simulink library "util_generic_model_lib"  (R2016b)
settings: Solver=ode45  StartTime=0.0  StopTime=10.0  RelTol=1e-3  EnableMultiTasking=on
undefined symbols (not defined in the file): abp_impeller_diameter, abp_impeller_speed2pwm, abp_nozzle_flap_count, abp_nozzle_flap_length, abp_nozzle_gear_ratio, abp_nozzle_intake_height, abp_nozzle_min_open_angle, abp_P_CG_B_B_error, abp_PM1_discharge_coeff, abp_pm1_impeller_orientation, abp_PM1_nozzle_orientations, abp_PM1_nozzle_widths, abp_PM1_P_nozzle_B_B, abp_pm1_zero_thrust_area, astrobee_time_step_size, bmp_PM1_impeller_orientation_error, bpm_imp_cmd_filt_den, bpm_imp_cmd_filt_num, bpm_imp_ctl_filt_n, bpm_imp_ctl_kd, bpm_imp_ctl_ki, bpm_imp_ctl_kp, bpm_imp_ctl_ts, bpm_imp_max_voltage, bpm_imp_motor_friction_coeff, bpm_imp_motor_r, bpm_imp_motor_speed_k, bpm_imp_motor_torque_k, bpm_imp_speed_filt_den, bpm_imp_speed_filt_num, bpm_impeller_inertia, bpm_impeller_inertia_error, bpm_impeller_init_speed, bpm_lookup_Cdp_data, bpm_lookup_totalarea_breakpoints, bpm_noise_on_flag, bpm_PM1_nozzle_discharge_coeff_error, bpm_PM1_nozzle_noise_feedback_gain, bpm_PM1_nozzle_thrust_noise_1s, bpm_PM1_P_nozzle_B_B_error, bpm_PM1_Q_nozzle2misaligned, bpm_PM1_randn_noise_seed, bpm_PM1_zero_thrust_area_error, bpm_sensor_delay, bpm_sensor_max, bpm_sensor_min, bpm_sensor_rand_seed, bpm_sensor_resolution, bpm_sensor_sf, bpm_sensor_sigma_u, bpm_sensor_sigma_v, bpm_servo_ctl_filt_n, bpm_servo_ctl_kd, bpm_servo_ctl_ki, bpm_servo_ctl_kp, bpm_servo_ctl_ts, bpm_servo_max_theta, bpm_servo_max_voltage, bpm_servo_min_theta, bpm_servo_motor_backlash_deadband ... (+45)
libraries: math_utils x8, simulink x4, vrlib x3, util_generic_model_lib x2
(part 1 of 2)
settings Model: Creator=rhnakamu  LastModifiedBy=jfusco1
settings DataIOCC: LimitDataPoints=on  SaveFormat=Array
settings OptimizationCC: LifeSpan=inf
settings DebuggingCC: AllowSymbolicDim=off  SFUnexpectedBacktrackingDiag=warning  SFNoUnconditionalDefaultTransitionDiag=warning  SFExecutionAtInitializationDiag=none
settings HardwareCC: ProdBitPerPointer=32  ProdBitPerSizeT=32  ProdBitPerPtrDiffT=32  ProdLargestAtomicFloat=None  ProdIntDivRoundTo=Undefined  ProdEndianess=Unspecified  ProdWordSize=32  ProdHWDeviceType=32-bit Generic
settings ModelReferenceCC: PropagateSignalLabelsOutOfModel=off
settings GRTTargetCC: TargetLangStandard=C89/C90 (ANSI)  GeneratePreprocessorConditionals=Disable all
settings ConfigComp: CovMetricSettings=dw  CovHtmlReporting=on  CovSaveCumulativeToWorkspaceVar=on  CovSaveSingleToWorkspaceVar=on  CovExternalEMLEnable=off

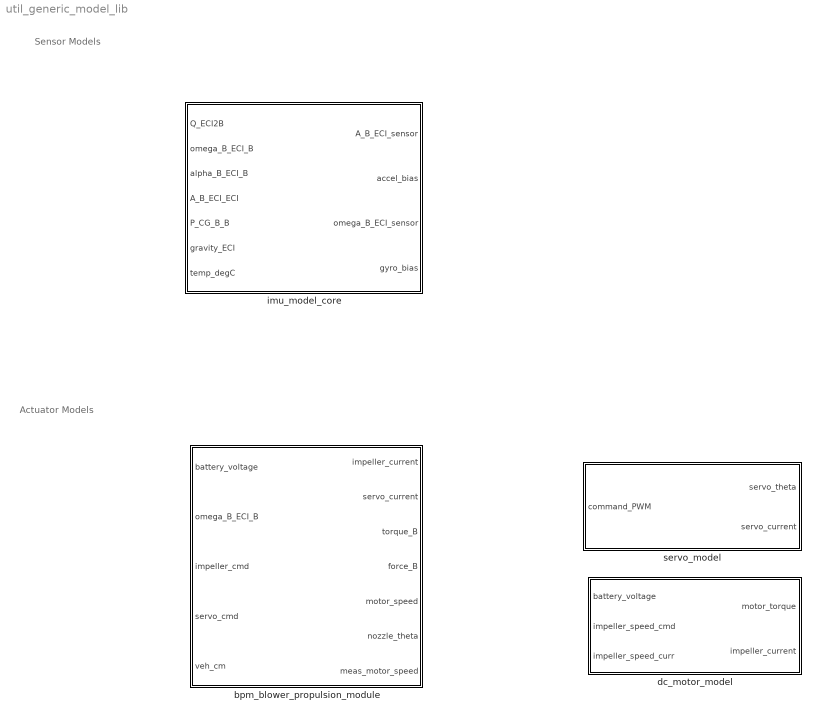
== system util_generic_model_lib ==
  note: Sensor Models
  note: Actuator Models
  bpm_blower_propulsion_module : Subsystem  mask{s_ctl_ts=bpm_servo_ctl_ts, s_ctl_pwm2angle=bpm_servo_pwm2angle, s_ctl_pwm2angle_bias=bpm_servo_pwm2angle_bias, s_ctl_kp=bpm_servo_ctl_kp, s_ctl_ki=bpm_servo_ctl_ki, s_ctl_kd=bpm_servo_ctl_kd, s_ctl_filt_n=bpm_servo_ctl_filt_n, s_ctl_max_volt=bpm_servo_max_voltage, s_motor_k=bpm_servo_motor_k, s_motor_r=bpm_servo_motor_r, s_motor_friction_coeff=bpm_servo_motor_friction_coeff, s_motor_gear_ratio=bpm_servo_motor_gear_ratio, s_motor_gear_box_inertia=bpm_servo_motor_gear_box_inertia, servo_max_theta=bpm_servo_max_theta, servo_min_theta=bpm_servo_min_theta, servo_backlash_deadband=bpm_servo_motor_backlash_deadband, P_nozzle_B_B=abp_PM1_P_nozzle_B_B, P_nozzle_B_B_offset=bpm_PM1_P_nozzle_B_B_error, nozzle_orientation_B=abp_PM1_nozzle_orientations, nozzle_orientation_offset=bpm_PM1_Q_nozzle2misaligned, noz_cd=abp_PM1_discharge_coeff, noz_cd_error=bpm_PM1_nozzle_discharge_coeff_error, noz_width=abp_PM1_nozzle_widths, noz_min_theta=abp_nozzle_min_open_angle, noz_intake_height=abp_nozzle_intake_height, noz_flap_length=abp_nozzle_flap_length, noz_flap_count=abp_nozzle_flap_count, noz_gear_ratio=abp_nozzle_gear_ratio, noz_thrust_noise=bpm_PM1_nozzle_thrust_noise_1s, noz_thrust_noise_feedback=bpm_PM1_nozzle_noise_feedback_gain, noz_randn_seed=bpm_PM1_randn_noise_seed, i_ctl_ts=bpm_imp_ctl_ts, i_ctl_pwm2speed=1/abp_impeller_speed2pwm, i_ctl_cmd_filt_num=bpm_imp_cmd_filt_num, i_ctl_cmd_filt_den=bpm_imp_cmd_filt_den, i_ctl_speed_filt_num=bpm_imp_speed_filt_num, i_ctl_speed_filt_den=bpm_imp_speed_filt_den, i_ctl_kp=bpm_imp_ctl_kp, i_ctl_ki=bpm_imp_ctl_ki, i_ctl_kd=bpm_imp_ctl_kd, i_ctl_filt_n=bpm_imp_ctl_filt_n, i_ctl_max_volt=bpm_imp_max_voltage, i_motor_kn=bpm_imp_motor_speed_k, i_motor_r=bpm_imp_motor_r, i_motor_kt=bpm_imp_motor_torque_k, i_motor_friction_coeff=bpm_imp_motor_friction_coeff, imp_unit_vec_B=abp_pm1_impeller_orientation, imp_unit_vec_B_offset=bmp_PM1_impeller_orientation_error, imp_zero_thrust_area=abp_pm1_zero_thrust_area, imp_zero_thrust_area_error=bpm_PM1_zero_thrust_area_error, imp_diameter=abp_impeller_diameter, imp_cdp_lookup=bpm_lookup_Cdp_data, imp_area_lookup=bpm_lookup_totalarea_breakpoints, imp_inertia=bpm_impeller_inertia, imp_inertia_error=bpm_impeller_inertia_error, imp_init_speed=bpm_impeller_init_speed, sens_sf=bpm_sensor_sf, sens_sigma_u=bpm_sensor_sigma_u, sens_sigma_v=bpm_sensor_sigma_v, sens_rand_seed=bpm_sensor_rand_seed, sens_resolution=bpm_sensor_resolution, sens_max=bpm_sensor_max, sens_min=bpm_sensor_min, sens_delay=bpm_sensor_delay, P_CG_B_B_error=abp_P_CG_B_B_error, const_air_den=const_air_density, sim_step_size=astrobee_time_step_size, noise_on_flag=bpm_noise_on_flag}
      mask prompts: s_ctl_ts "Controller Sample Time"; s_ctl_pwm2angle "PWM2Angle Conversion Gain"; s_ctl_pwm2angle_bias "PWM2Angle Conversion Bias"; s_ctl_kp "PID Controller - P gain"; s_ctl_ki "PID Controller - I gain"; s_ctl_kd "PID Controller - D gain"; s_ctl_filt_n "PID Controller - filter"; s_ctl_max_volt "Max Voltage Output"; s_motor_k "Speed Constant (k)"; s_motor_r "Resistance (r)"; s_motor_friction_coeff "Friction Coefficient"; s_motor_gear_ratio "Gear Ratio"; s_motor_gear_box_inertia "Gear Box Inertia"; servo_max_theta "Servo Max Theta"; servo_min_theta "Servo Min Theta"; servo_backlash_deadband "Backlash Deadband"; P_nozzle_B_B_offset "P_nozzle_B_B offset"; nozzle_orientation_B "Nozzle Orientation (B frame)"; nozzle_orientation_offset "Nozzle Orientation (offset)"; noz_cd "Discharge Coefficients"; noz_cd_error "Discharge Coefficients Error"; noz_width "Widths"; noz_min_theta "Min Theta"; noz_intake_height "Intake Height"; noz_flap_length "Flap Length"; noz_flap_count "Flap Count (per nozzle)"; noz_gear_ratio "Servo2Nozzle Gear Ratio"; noz_thrust_noise "Nozzle Thrust Noise (1-sigma)"; noz_thrust_noise_feedback "Nozzle Thrust Noise Feedback Gain"; noz_randn_seed "Nozzle Randn Seed"; i_ctl_ts "Controller Sample Time"; i_ctl_pwm2speed "PWM2Speed Conversion Gain"; i_ctl_cmd_filt_num "Speed Cmd Filter (Num)"; i_ctl_cmd_filt_den "Speed Cmd Filter (Den)"; i_ctl_speed_filt_num "Speed Filt (Num)"; i_ctl_speed_filt_den "Speed Filt (Den)"; i_ctl_kp "PID Controller - P gain"; i_ctl_ki "PID Controller - I Gain"; i_ctl_kd "PID Controller - D gain"; i_ctl_filt_n "PID Controller - filter"; i_ctl_max_volt "Max Voltage Output"; i_motor_kn "Speed Constant (kn)"; i_motor_r "Resistance (r)"; i_motor_kt "Torque Constant (kt)"; i_motor_friction_coeff "Friction Coefficient"; imp_unit_vec_B "Rotational Unit Vector (B frame)"; imp_unit_vec_B_offset "Rotational Unit Vector Offset"; imp_zero_thrust_area "Zero Thrust Area (Leakage)"; imp_zero_thrust_area_error "Zero Thrust Area Error"; imp_diameter "Diameter"; imp_cdp_lookup "Lookup Cdp data"; imp_area_lookup "Lookup totalarea breakpoints"; imp_inertia "Inertia"; imp_inertia_error "Inertia Error"; imp_init_speed "Initial Speed"; sens_sf "Scale Factor"; sens_sigma_u "Sigma U (noise)"; sens_sigma_v "Sigma V (noise)"; sens_rand_seed "Randn Seed"; sens_resolution "Resolution"; sens_max "Max Output"; sens_min "Min Output"; sens_delay "Output Delay"; P_CG_B_B_error "Position of CG error"; const_air_den "Air Density Constant"; sim_step_size "Simulation Step Size"; noise_on_flag "Noise On Flag (1=on, 0=off)"
      mask DialogControl DescGroupVar Prompt: Blower Propulsion Model Parameters
  dc_motor_model : Subsystem  mask{controller_sample_time=0, ctl_pwm2speed=0, ctl_cmd_filt_num=0, ctl_cmd_filt_den=0, ctl_speed_filt_num=0, ctl_speed_cilt_den=0, ctl_kp=0, ctl_ki=0, ctl_kd=0, ctl_filt_n=0, ctl_max_voltage=0, motor_kn=0, motor_r=0, motor_kt=0, motor_friction_coeff=0}
      mask prompts: controller_sample_time "Controller Sample Time"; ctl_pwm2speed "PWM2Speed Conversion Gain"; ctl_cmd_filt_num "Speed Cmd Filter (Num)"; ctl_cmd_filt_den "Speed Cmd Filter (Den)"; ctl_speed_filt_num "Speed Filter (Num)"; ctl_speed_cilt_den "Speed Filter (Den)"; ctl_kp "PID Controller - P Gain"; ctl_ki "PID Controller - I Gain"; ctl_kd "PID Controller - D Gain"; ctl_filt_n "PID Controller - filter"; ctl_max_voltage "Max Voltage Output"; motor_kn "Speed Constant (kn)"; motor_r "Resistance (r)"; motor_kt "Torque Constant (kt)"; motor_friction_coeff "Friction Coefficient"
      mask DialogControl DescGroupVar Prompt: Generic DC Motor Model
  imu_model_core : Subsystem  mask{Q_B2accel_nominal=epson_Q_B2accel, Q_B2accel_error=0, Q_B2gyro_nominal=epson_Q_B2gyro, Q_B2gyro_error=0, P_sensor_B_B_nominal=epson_P_sensor_B_B, P_sensor_B_B_error=0, imu_output_delay=epson_output_delay, sample_time=astrobee_time_step_size, report_imu_truth=epson_gyro_report_truth, no_rot_effects=epson_no_rot_effects, accel_sf=epson_accel_sf_coef, accel_nonlinear_coeff=epson_accel_nonlinearity_coeff, accel_temp_coeff=epson_accel_temp_bias_coeff, accel_sigma_vrw=epson_accel_sigma_v, accel_sigma_arw=epson_accel_sigma_u, accel_bias_ic=epson_accel_bias_ic, accel_sigma_markov=epson_accel_sigma_w, accel_markov_tau=epson_accel_markov_tau, accel_noise_seed=epson_accel_noise_seed, accel_filter_num=epson_accel_filt_num, accel_filter_den=epson_accel_filt_den, accel_resolution=epson_accel_resolution, accel_upper_sat=epson_accel_upper_sat, accel_lower_sat=epson_accel_lower_sat, gyro_sf=epson_gyro_sf_coef, gyro_accel_sensitivity=epson_gyro_linear_accel_bias_coeff, gyro_nonlinear_coeff=epson_gyro_nonlinearity_coeff, gyro_temp_coeff=epson_gyro_temp_bias_coeff, gyro_sigma_arw=epson_gyro_sigma_v, gyro_sigma_rrw=epson_gyro_sigma_u, gyro_bias_ic=epson_gyro_bias_ic, gyro_sigma_markov=epson_gyro_sigma_w, gyro_markov_tau=epson_gyro_markov_tau, gyro_noise_seed=epson_gyro_noise_seed, gyro_filter_num=epson_gyro_filt_num, gyro_filter_den=epson_gyro_filt_den, gyro_resolution=epson_gyro_resolution, gyro_upper_sat=epson_gyro_upper_sat, gyro_lower_sat=epson_gyro_lower_sat}
      mask prompts: Q_B2accel_nominal "Q_B2accel (nominal):"; Q_B2accel_error "Q_B2accel (errors):"; Q_B2gyro_nominal "Q_B2gyro (nominal):"; Q_B2gyro_error "Q_B2gyro (errors):"; P_sensor_B_B_nominal "P_sensor_B_B (nominal):"; P_sensor_B_B_error "P_sensor_B_B (error):"; imu_output_delay "Output Delay:"; sample_time "Sample Time:"; report_imu_truth "Report Truth Flag"; no_rot_effects "No Rot Effects Flag"; accel_sf "Scale Factor Coefficient:"; accel_nonlinear_coeff "Non Linearity Coefficient:"; accel_temp_coeff "Temperature Coefficient:"; accel_sigma_vrw "Velocity Random Walk Sigma (m/s^(3/2))"; accel_sigma_arw "Acceleration Random Walk Sigma (m/sec^(5/2))"; accel_bias_ic "Bias I.C."; accel_sigma_markov "Markov Random Drift ((m/s^2)/s)"; accel_markov_tau "Markov Tau constant"; accel_noise_seed "Random Number Seed"; accel_filter_num "Internal Filter Numerator (coefficients)"; accel_filter_den "Internal Filter Denominator (coefficients)"; accel_resolution "Resolution:"; accel_upper_sat "Upper Saturation:"; accel_lower_sat "Lower Saturation:"; gyro_sf "Scale Factor Coefficient:"; gyro_accel_sensitivity "Linear Accel Coefficient:"; gyro_nonlinear_coeff "Non Linearity Coefficient:"; gyro_temp_coeff "Temperature Coefficient:"; gyro_sigma_arw "Angular Random Walk Sigma (rad/sqrt(sec))"; gyro_sigma_rrw "Rate Random Walk Sigma (rad/sec^(3/2))"; gyro_bias_ic "Bias I.C."; gyro_sigma_markov "Markov Random Drift (deg/s)"; gyro_markov_tau "Markov Tau Constant"; gyro_noise_seed "Random Number Seed"; gyro_filter_num "Internal Filter Numerator (coefficients)"; gyro_filter_den "Internal Filter Denominator (coefficients)"; gyro_resolution "Resolution:"; gyro_upper_sat "Upper Saturation:"; gyro_lower_sat "Lower Saturation:"
      mask DialogControl DescTextVar Prompt: Properties for the generic IMU model.
      mask DialogControl Container25 Prompt: Debugging Properties
      mask DialogControl Control6 Prompt: Units are m/s^2 unless stated
      mask DialogControl Container17 Prompt: Scale Factor
      mask DialogControl Container19 Prompt: Bias Coefficients:
      mask DialogControl Container16 Prompt: Noise Parameters
      mask DialogControl Container18 Prompt: Hardware Properties
      mask DialogControl Control7 Prompt: Units are rad/sec unless stated
      mask DialogControl Container20 Prompt: Scale Factor:
      mask DialogControl Container21 Prompt: Bias Coefficients:
      mask DialogControl Container16_copy_copy Prompt: Noise Parameters
      mask DialogControl Container18_copy Prompt: Hardware Properties
  servo_model : Subsystem  TreatAsAtomicUnit=on  mask{controller_sample_time=0, servo_pwm2angle=0, servo_pwm2angle_bias=0, servo_ctl_kp=0, servo_ctl_ki=0, servo_ctl_kd=0, servo_ctl_filt_n=0, servo_ctl_ts=0, servo_max_voltage=0, motor_k=0, motor_r=0, motor_friction_coeff=0, motor_gear_ratio=0, motor_gear_box_inertia=0, servo_max_theta=0, servo_min_theta=0, motor_backlash_deadband=0}
      mask prompts: controller_sample_time "Controller Sample Time"; servo_pwm2angle "PWM2Angle Conversion Gain"; servo_pwm2angle_bias "PWM2Angle Conversion Bias"; servo_ctl_kp "PID Controller - P gain"; servo_ctl_ki "PID Controller - I gain"; servo_ctl_kd "PID Controller - D gain"; servo_ctl_filt_n "PID Controller - filter"; servo_ctl_ts "PID Controller - sample time"; servo_max_voltage "Max Voltage output"; motor_k "Speed Constant (k)"; motor_r "Resistance (r)"; motor_friction_coeff "Friction Coefficient"; motor_gear_ratio "Gear Ratio"; motor_gear_box_inertia "Gear Box Inertia"; servo_max_theta "Servo Max Theta"; servo_min_theta "Servo Min Theta"; motor_backlash_deadband "Backlash Deadband"
      mask DialogControl DescGroupVar Prompt: Generic Servo Model

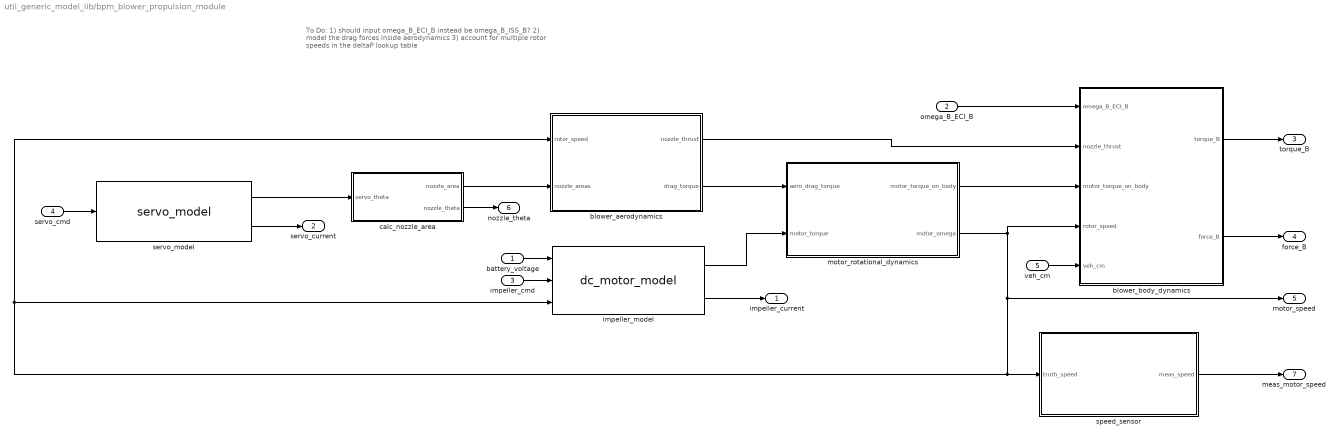
== system util_generic_model_lib/bpm_blower_propulsion_module ==
  note: To Do:
      | 	1) should input omega_B_ECI_B instead be omega_B_ISS_B?
      | 	2) model the drag forces inside aerodynamics
      | 	3) account for multiple rotor speeds in the deltaP lookup table
  battery_voltage : Inport
  omega_B_ECI_B : Inport  Port=2
  impeller_cmd : Inport  Port=3
  servo_cmd : Inport  Port=4
  veh_cm : Inport  Port=5
  blower_aerodynamics : Subsystem  TreatAsAtomicUnit=on  VariantControl=blw_blower_algebraic == true
      settings: RTWFcnNameOpts=Use subsystem name  RTWFileNameOpts=Use subsystem name
  blower_body_dynamics : Subsystem
  calc_nozzle_area : Subsystem  TreatAsAtomicUnit=on
  impeller_model : util_generic_model_lib/dc_motor_model  controller_sample_time=i_ctl_ts  ctl_pwm2speed=i_ctl_pwm2speed  ctl_cmd_filt_num=i_ctl_cmd_filt_num  ctl_cmd_filt_den=i_ctl_cmd_filt_den  ctl_speed_filt_num=i_ctl_speed_filt_num  ctl_speed_cilt_den=i_ctl_speed_filt_den  ctl_kp=i_ctl_kp  ctl_ki=i_ctl_ki  ctl_kd=i_ctl_kd  ctl_filt_n=i_ctl_filt_n  ctl_max_voltage=i_ctl_max_volt  motor_kn=i_motor_kn  motor_r=i_motor_r  motor_kt=i_motor_kt  motor_friction_coeff=i_motor_friction_coeff
  motor_rotational_dynamics : Subsystem
  servo_model : util_generic_model_lib/servo_model  controller_sample_time=s_ctl_ts  servo_pwm2angle=s_ctl_pwm2angle  servo_pwm2angle_bias=s_ctl_pwm2angle_bias  servo_ctl_kp=s_ctl_kp  servo_ctl_ki=s_ctl_ki  servo_ctl_kd=s_ctl_kd  servo_ctl_filt_n=s_ctl_filt_n  servo_ctl_ts=s_ctl_ts  servo_max_voltage=s_ctl_max_volt  motor_k=s_motor_k  motor_r=s_motor_r  motor_friction_coeff=s_motor_friction_coeff  motor_gear_ratio=s_motor_gear_ratio  motor_gear_box_inertia=s_motor_gear_box_inertia  servo_max_theta=servo_max_theta  servo_min_theta=servo_min_theta  motor_backlash_deadband=servo_backlash_deadband
  speed_sensor : Subsystem
  impeller_current : Outport
  servo_current : Outport  Port=2
  torque_B : Outport  Port=3
  force_B : Outport  Port=4
  motor_speed : Outport  Port=5
  nozzle_theta : Outport  Port=6
  meas_motor_speed : Outport  Port=7
  wires:
  blower_aerodynamics/1(nozzle_thrust) -> blower_body_dynamics/2(nozzle_thrust)
  battery_voltage/1 -> impeller_model/1
  calc_nozzle_area/1(nozzle_area) -> blower_aerodynamics/2(nozzle_areas)
  motor_rotational_dynamics/2(motor_omega) -> blower_body_dynamics/4(rotor_speed), motor_speed/1, impeller_model/3, blower_aerodynamics/1(rotor_speed), speed_sensor/1(truth_speed)
  servo_model/2 -> servo_current/1
  speed_sensor/1(meas_speed) -> meas_motor_speed/1
  omega_B_ECI_B/1 -> blower_body_dynamics/1(omega_B_ECI_B)
  servo_cmd/1 -> servo_model/1
  impeller_cmd/1 -> impeller_model/2
  impeller_model/1 -> motor_rotational_dynamics/2(motor_torque)
  impeller_model/2 -> impeller_current/1
  blower_aerodynamics/2(drag_torque) -> motor_rotational_dynamics/1(aero_drag_torque)
  motor_rotational_dynamics/1(motor_torque_on_body) -> blower_body_dynamics/3(motor_torque_on_body)
  servo_model/1 -> calc_nozzle_area/1(servo_theta)
  calc_nozzle_area/2(nozzle_theta) -> nozzle_theta/1
  blower_body_dynamics/1(torque_B) -> torque_B/1
  blower_body_dynamics/2(force_B) -> force_B/1
  veh_cm/1 -> blower_body_dynamics/5(veh_cm)

== system util_generic_model_lib/dc_motor_model ==
  battery_voltage : Inport
  impeller_speed_cmd : Inport  Port=2
  impeller_speed_curr : Inport  Port=3
  Rate Transition1 : RateTransition  OutPortSampleTime=controller_sample_time
      settings: AttributesFormatString=sampleTime: %<OutPortSampleTime>
  Rate Transition2 : RateTransition  OutPortSampleTime=controller_sample_time
      settings: AttributesFormatString=sampleTime: %<OutPortSampleTime>
  Rate Transition3 : RateTransition
      settings: AttributesFormatString=sampleTime: %<OutPortSampleTime>
  Rate Transition4 : RateTransition  OutPortSampleTime=controller_sample_time
      settings: AttributesFormatString=sampleTime: %<OutPortSampleTime>
  dc_motor_model : Subsystem  TreatAsAtomicUnit=on
  speed_controller : Subsystem  TreatAsAtomicUnit=on
  motor_torque : Outport
  impeller_current : Outport  Port=2
  wires:
  impeller_speed_curr/1 -> Rate Transition4/1, dc_motor_model/2(curr_rotor_speed)
  dc_motor_model/1(motor_torque) -> motor_torque/1
  speed_controller/1(motor_ctl_voltage) -> Rate Transition3/1
  dc_motor_model/2(motor_current) -> impeller_current/1
  battery_voltage/1 -> Rate Transition1/1
  Rate Transition3/1 -> dc_motor_model/1(ctl_voltage)
  Rate Transition1/1 -> speed_controller/1(battery_voltage)
  Rate Transition2/1 -> speed_controller/2(speed_cmd)
  Rate Transition4/1 -> speed_controller/3(speed_curr)
  impeller_speed_cmd/1 -> Rate Transition2/1

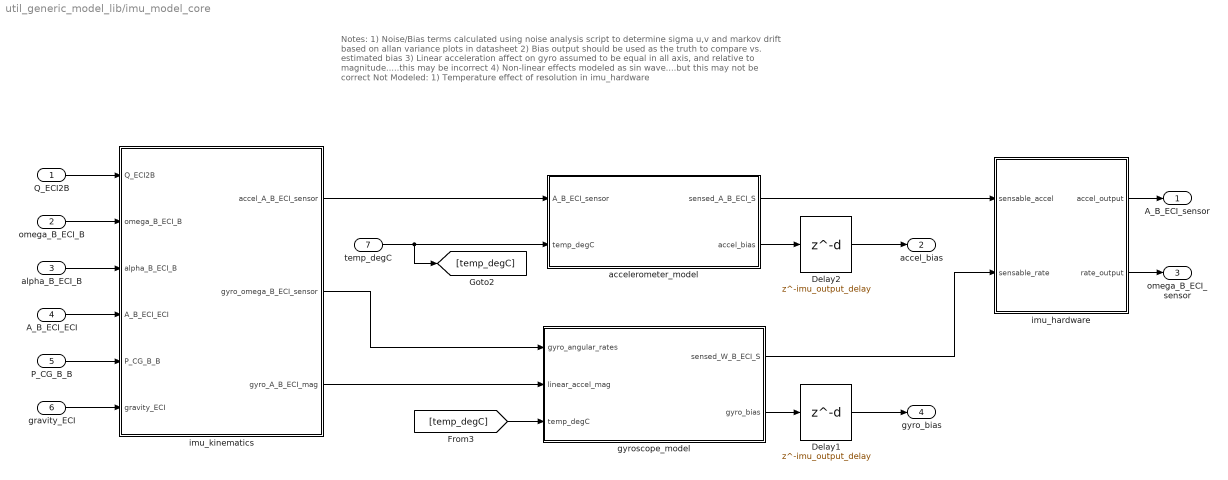
== system util_generic_model_lib/imu_model_core ==
  note: Notes:
      | 	1) Noise/Bias terms calculated using noise analysis script to determine sigma u,v and markov drift based on allan variance plots in datasheet
      | 	2) Bias output should be used as the truth to compare vs. estimated bias
      | 	3) Linear acceleration affect on gyro assumed to be equal in all axis, and relative to magnitude.....this may be incorrect
      | 	4) Non-linear effects modeled as sin wave....but this may not be correct
      |
      | Not Modeled:
      | 	1) Temperature effect of resolution in imu_hardware
  Q_ECI2B : Inport
  omega_B_ECI_B : Inport  Port=2
  alpha_B_ECI_B : Inport  Port=3
  A_B_ECI_ECI : Inport  Port=4
  P_CG_B_B : Inport  Port=5
  gravity_ECI : Inport  Port=6
  temp_degC : Inport  Port=7
  Delay1 : Delay  DelayLength=imu_output_delay
      settings: AttributesFormatString=|
      | IC: %<InitialCondition>
      | Delay: %<DelayLength>
  Delay2 : Delay  DelayLength=imu_output_delay
      settings: AttributesFormatString=|
      | IC: %<InitialCondition>
      | Delay: %<DelayLength>
  accelerometer_model : Subsystem
  gyroscope_model : Subsystem
  imu_hardware : Subsystem
  imu_kinematics : Subsystem
  A_B_ECI_sensor : Outport
  accel_bias : Outport  Port=2
  omega_B_ECI_sensor : Outport  Port=3
  gyro_bias : Outport  Port=4
  wires:
  omega_B_ECI_B/1 -> imu_kinematics/2(omega_B_ECI_B)
  imu_kinematics/2(gyro_omega_B_ECI_sensor) -> gyroscope_model/1(gyro_angular_rates)
  Delay1/1 -> gyro_bias/1
  Delay2/1 -> accel_bias/1
  [temp_degC] -> gyroscope_model/3(temp_degC)
  temp_degC/1 -> accelerometer_model/2(temp_degC), [temp_degC]
  imu_kinematics/1(accel_A_B_ECI_sensor) -> accelerometer_model/1(A_B_ECI_sensor)
  imu_kinematics/3(gyro_A_B_ECI_mag) -> gyroscope_model/2(linear_accel_mag)
  accelerometer_model/1(sensed_A_B_ECI_S) -> imu_hardware/1(sensable_accel)
  gyroscope_model/1(sensed_W_B_ECI_S) -> imu_hardware/2(sensable_rate)
  alpha_B_ECI_B/1 -> imu_kinematics/3(alpha_B_ECI_B)
  Q_ECI2B/1 -> imu_kinematics/1(Q_ECI2B)
  A_B_ECI_ECI/1 -> imu_kinematics/4(A_B_ECI_ECI)
  P_CG_B_B/1 -> imu_kinematics/5(P_CG_B_B)
  gravity_ECI/1 -> imu_kinematics/6(gravity_ECI)
  imu_hardware/2(rate_output) -> omega_B_ECI_sensor/1
  imu_hardware/1(accel_output) -> A_B_ECI_sensor/1
  gyroscope_model/2(gyro_bias) -> Delay1/1
  accelerometer_model/2(accel_bias) -> Delay2/1

== system util_generic_model_lib/servo_model ==
  command_PWM : Inport
  Rate Transition1 : RateTransition  OutPortSampleTime=controller_sample_time
      settings: AttributesFormatString=sampleTime: %<OutPortSampleTime>
  Rate Transition2 : RateTransition  OutPortSampleTime=controller_sample_time
      settings: AttributesFormatString=sampleTime: %<OutPortSampleTime>
  Rate Transition3 : RateTransition
      settings: AttributesFormatString=sampleTime: %<OutPortSampleTime>
  Terminator : Terminator
  dc_motor_dynamics : Subsystem
  servo_controller : Subsystem
  servo_theta : Outport
  servo_current : Outport  Port=2
  wires:
  dc_motor_dynamics/1(servo_theta) -> Rate Transition2/1, servo_theta/1
  dc_motor_dynamics/2(servo_current) -> servo_current/1
  Rate Transition2/1 -> servo_controller/2(curr_servo_theta)
  Rate Transition1/1 -> servo_controller/1(command_PWM)
  Rate Transition3/1 -> dc_motor_dynamics/1(ctl_voltage)
  servo_controller/1(motor_ctl_voltage) -> Rate Transition3/1
  command_PWM/1 -> Rate Transition1/1
  dc_motor_dynamics/3(servo_torque) -> Terminator/1

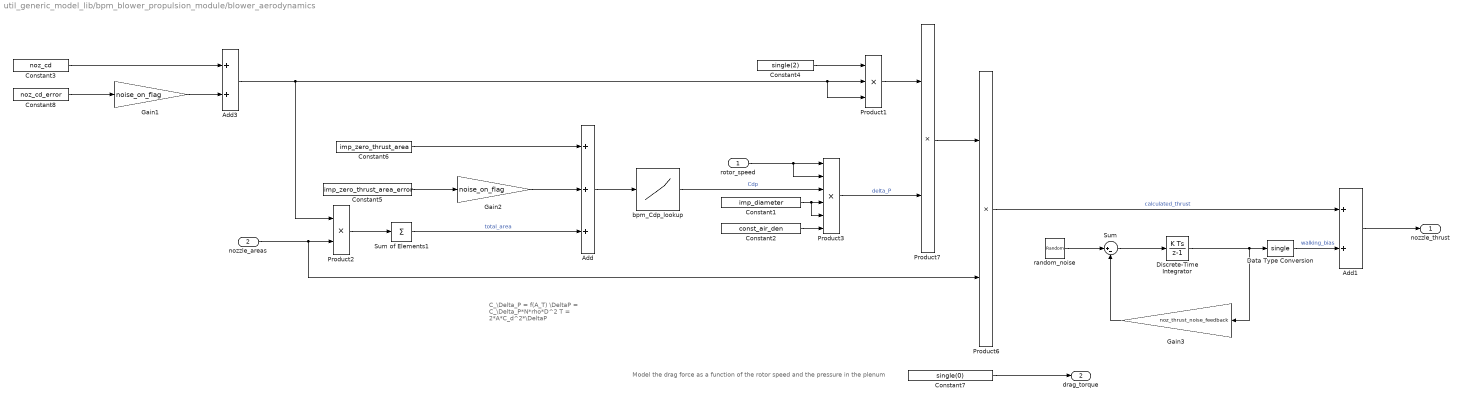
== system util_generic_model_lib/bpm_blower_propulsion_module/blower_aerodynamics ==
  note: Model the drag force as a function of the rotor speed and the pressure in the plenum
  note: C_\Delta_P = f(A_T)
      | \DeltaP = C_\Delta_P*N*rho*D^2
      | T = 2*A*C_d^2*\DeltaP
  rotor_speed : Inport
  nozzle_areas : Inport  Port=2
  Add : Sum  Inputs=+++
  Add1 : Sum
  Add3 : Sum
  Constant1 : Constant  Value=imp_diameter
  Constant2 : Constant  Value=const_air_den
  Constant3 : Constant  Value=noz_cd
  Constant4 : Constant  Value=single(2)
  Constant5 : Constant  Value=imp_zero_thrust_area_error
  Constant6 : Constant  Value=imp_zero_thrust_area
  Constant7 : Constant  Value=single(0)
  Constant8 : Constant  Value=noz_cd_error
  Data Type Conversion : DataTypeConversion  OutDataTypeStr=single
  Discrete-Time Integrator : DiscreteIntegrator  InitialConditionSetting=State (most efficient)  SampleTime=-1  ICPrevOutput=DiscIntNeverNeededParam  ICPrevScaledInput=DiscIntNeverNeededParam
      settings: AttributesFormatString=IC:%<InitialCondition>
  Gain1 : Gain  Gain=noise_on_flag
  Gain2 : Gain  Gain=noise_on_flag
  Gain3 : Gain  Gain=noz_thrust_noise_feedback
  Product1 : Product  Inputs=***
  Product2 : Product  Inputs=**
  Product3 : Product  Inputs=******
  Product6 : Product  Inputs=**
  Product7 : Product  Inputs=**
  Sum : Sum  Inputs=|+-
  Sum of Elements1 : Sum  Inputs=+
  bpm_Cdp_lookup : Lookup_n-D  NumberOfTableDimensions=1  BreakpointsForDimension1=imp_area_lookup  BreakpointsForDimension3=[5, 7]  Table=imp_cdp_lookup  InternalRulePriority=Speed  RndMeth=Simplest  InputSameDT=on
      settings: AttributesFormatString=|
      | data table: %<Table>
      | #dim: %<NumberOfTableDimensions>
      | BP1: %<BreakpointsForDimension1>
  random_noise : RandomNumber  Variance=noz_thrust_noise.^2  Seed=noz_randn_seed +[1:6]  SampleTime=sim_step_size
      settings: AttributesFormatString=|
      | Variance:%<Variance>
      | Mean:%<Mean>
      | Seed:%<Seed>
      | Sample Time:%<SampleTime>
  nozzle_thrust : Outport
  drag_torque : Outport  Port=2
  wires:
  Data Type Conversion/1 -> Add1/2  "walking_bias"
  Add1/1 -> nozzle_thrust/1
  Product6/1 -> Add1/1  "calculated_thrust"
  Gain3/1 -> Sum/2
  random_noise/1 -> Sum/1
  Sum/1 -> Discrete-Time Integrator/1
  Discrete-Time Integrator/1 -> Gain3/1, Data Type Conversion/1
  Constant2/1 -> Product3/6
  Product3/1 -> Product7/2  "delta_P"
  Constant1/1 -> Product3/5, Product3/4
  nozzle_areas/1 -> Product2/2, Product6/2
  Product1/1 -> Product7/1
  Constant4/1 -> Product1/1
  Add3/1 -> Product1/2, Product1/3, Product2/1
  bpm_Cdp_lookup/1 -> Product3/3  "Cdp"
  Sum of Elements1/1 -> Add/3  "total_area"
  rotor_speed/1 -> Product3/1, Product3/2
  Constant7/1 -> drag_torque/1
  Add/1 -> bpm_Cdp_lookup/1
  Constant6/1 -> Add/1
  Product2/1 -> Sum of Elements1/1
  Product7/1 -> Product6/1
  Constant8/1 -> Gain1/1
  Gain1/1 -> Add3/2
  Constant3/1 -> Add3/1
  Constant5/1 -> Gain2/1
  Gain2/1 -> Add/2

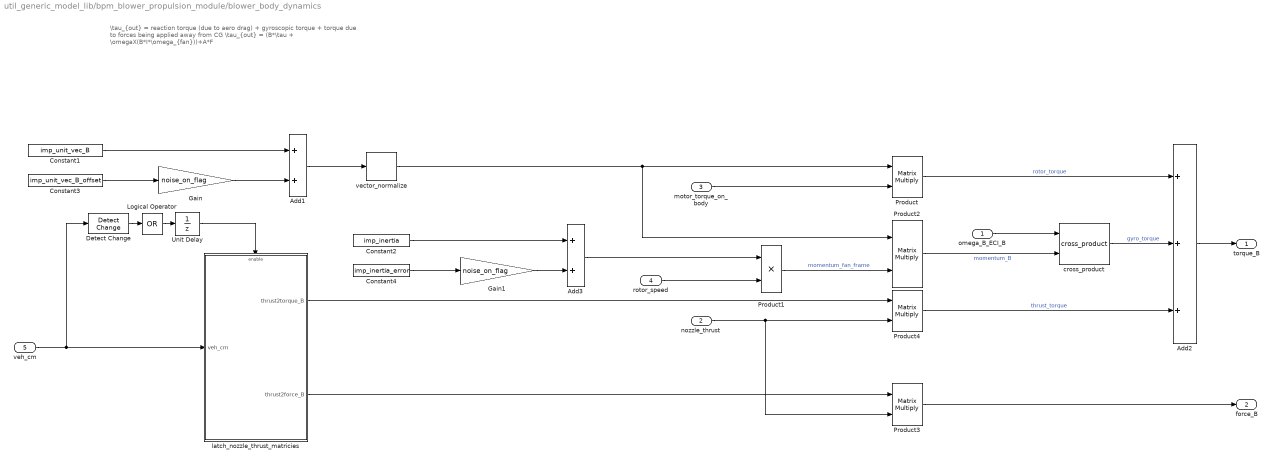
== system util_generic_model_lib/bpm_blower_propulsion_module/blower_body_dynamics ==
  note: \tau_{out} = reaction torque (due to aero drag)
      |                      + gyroscopic torque
      |                      + torque due to forces being applied away from CG
      | \tau_{out} = (B*\tau + \omegaX(B*I*\omega_{fan}))+A*F
  omega_B_ECI_B : Inport
  nozzle_thrust : Inport  Port=2
  motor_torque_on_body : Inport  Port=3
  rotor_speed : Inport  Port=4
  veh_cm : Inport  Port=5
  Add1 : Sum
  Add2 : Sum  Inputs=+++
  Add3 : Sum
  Constant1 : Constant  Value=imp_unit_vec_B
  Constant2 : Constant  Value=imp_inertia
  Constant3 : Constant  Value=imp_unit_vec_B_offset
  Constant4 : Constant  Value=imp_inertia_error
  Detect Change : simulink/Logic and Bit Operations/Detect Change  vinit=0  OutDataTypeStr=boolean
  Gain : Gain  Gain=noise_on_flag
  Gain1 : Gain  Gain=noise_on_flag
  Logical Operator : Logic  Operator=OR  Inputs=1  AllPortsSameDT=off  OutDataTypeStr=boolean
  Product{,2..4} (4 alike) : Product  Multiplication=Matrix(*)
  Product1 : Product
  Unit Delay : UnitDelay  InitialCondition=1  SampleTime=-1
      settings: AttributesFormatString=IC: %<InitialCondition>
  cross_product : math_utils/cross_product  SystemSampleTime=-1
  latch_nozzle_thrust_matricies : Subsystem
  vector_normalize : math_utils/vector_normalize  SystemSampleTime=-1
  torque_B : Outport
  force_B : Outport  Port=2
  wires:
  vector_normalize/1 -> Product2/1, Product/1
  Logical Operator/1 -> Unit Delay/1
  Unit Delay/1 -> latch_nozzle_thrust_matricies/Enable
  Product4/1 -> Add2/3  "thrust_torque"
  Product3/1 -> force_B/1
  nozzle_thrust/1 -> Product3/2, Product4/2
  Add2/1 -> torque_B/1
  cross_product/1 -> Add2/2  "gyro_torque"
  Product/1 -> Add2/1  "rotor_torque"
  Product2/1 -> cross_product/2  "momentum_B"
  omega_B_ECI_B/1 -> cross_product/1
  Product1/1 -> Product2/2  "momentum_fan_frame"
  Add1/1 -> vector_normalize/1
  rotor_speed/1 -> Product1/2
  motor_torque_on_body/1 -> Product/2
  Constant1/1 -> Add1/1
  Constant3/1 -> Gain/1
  Gain/1 -> Add1/2
  Constant4/1 -> Gain1/1
  Gain1/1 -> Add3/2
  Constant2/1 -> Add3/1
  Add3/1 -> Product1/1
  latch_nozzle_thrust_matricies/1(thrust2torque_B) -> Product4/1
  latch_nozzle_thrust_matricies/2(thrust2force_B) -> Product3/1
  veh_cm/1 -> Detect Change/1, latch_nozzle_thrust_matricies/1(veh_cm)
  Detect Change/1 -> Logical Operator/1

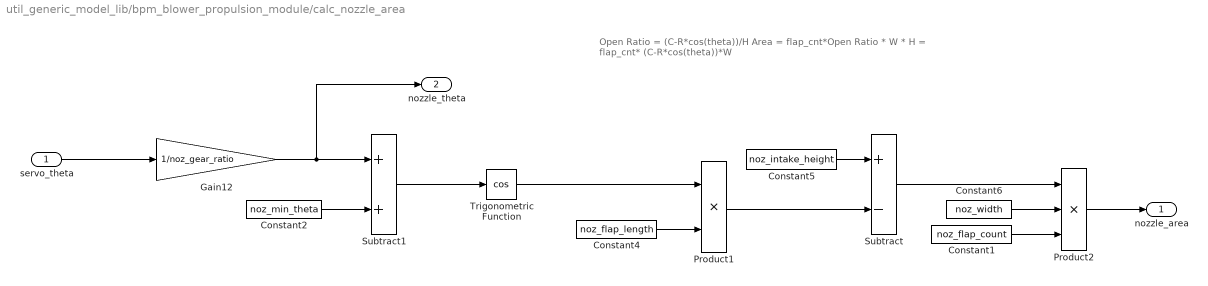
== system util_generic_model_lib/bpm_blower_propulsion_module/calc_nozzle_area ==
  note: Open Ratio = (C-R*cos(theta))/H
      |
      | Area = flap_cnt*Open Ratio * W * H = flap_cnt* (C-R*cos(theta))*W
  servo_theta : Inport
  Constant1 : Constant  Value=noz_flap_count
  Constant2 : Constant  Value=noz_min_theta
  Constant4 : Constant  Value=noz_flap_length
  Constant5 : Constant  Value=noz_intake_height
  Constant6 : Constant  Value=noz_width
  Gain12 : Gain  Gain=1/noz_gear_ratio
  Product1 : Product  Inputs=**
  Product2 : Product  Inputs=***
  Subtract : Sum  Inputs=+-
  Subtract1 : Sum
  Trigonometric Function : Trigonometry  Operator=cos
      settings: AttributesFormatString=Approx Method: %<ApproximationMethod>
  nozzle_area : Outport
  nozzle_theta : Outport  Port=2
  wires:
  Trigonometric Function/1 -> Product1/1
  Constant4/1 -> Product1/2
  Product1/1 -> Subtract/2
  Constant5/1 -> Subtract/1
  Subtract/1 -> Product2/1
  Constant6/1 -> Product2/2
  Constant1/1 -> Product2/3
  Subtract1/1 -> Trigonometric Function/1
  Product2/1 -> nozzle_area/1
  Constant2/1 -> Subtract1/2
  Gain12/1 -> Subtract1/1, nozzle_theta/1
  servo_theta/1 -> Gain12/1

== system util_generic_model_lib/bpm_blower_propulsion_module/motor_rotational_dynamics ==
  note: \tau_{total} = J*\omega' = \tau_{motor} -\tau_{drag} - \tau_{friction}
      |
      | Note: \tau_{friction} is accounted for in the motor model
  aero_drag_torque : Inport
  motor_torque : Inport  Port=2
  Add : Sum  Inputs=+-
  Constant : Constant  Value=noise_on_flag
  Discrete-Time Integrator : DiscreteIntegrator  InitialCondition=imp_init_speed  SampleTime=sim_step_size  ICPrevOutput=DiscIntNeverNeededParam  ICPrevScaledInput=DiscIntNeverNeededParam
      settings: AttributesFormatString=|
      | IC: %<InitialCondition>
      | TS: %<SampleTime>
  Gain : Gain  Gain=1./imp_inertia
  Gain1 : Gain  Gain=-1
  Gain2 : Gain  Gain=1./(imp_inertia+imp_inertia_error)
  Switch : Switch  Criteria=u2 > Threshold
  motor_torque_on_body : Outport
  motor_omega : Outport  Port=2
  wires:
  Discrete-Time Integrator/1 -> motor_omega/1  "omega"
  Gain1/1 -> motor_torque_on_body/1  "torque_on_body_due_to_motor"
  Add/1 -> Gain/1, Gain2/1  "torque_on_motor"
  Switch/1 -> Discrete-Time Integrator/1  "omega_dot"
  motor_torque/1 -> Gain1/1, Add/1
  aero_drag_torque/1 -> Add/2
  Constant/1 -> Switch/2
  Gain/1 -> Switch/1
  Gain2/1 -> Switch/3

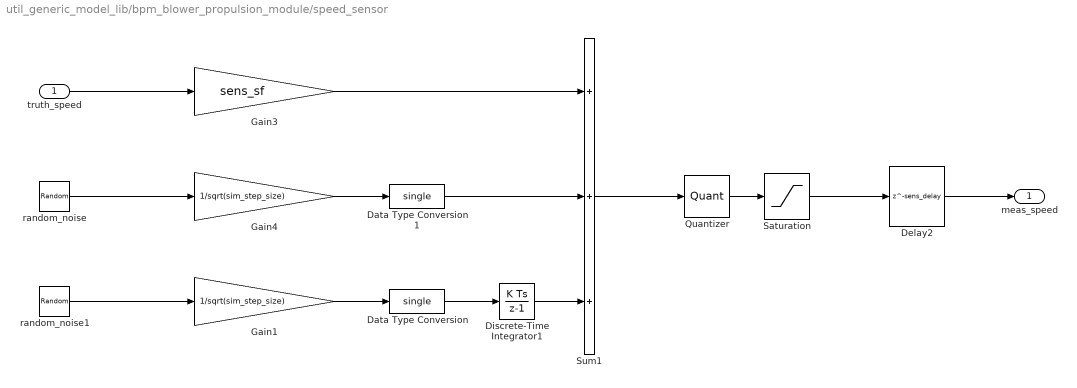
== system util_generic_model_lib/bpm_blower_propulsion_module/speed_sensor ==
  truth_speed : Inport
  Data Type Conversion : DataTypeConversion  OutDataTypeStr=single
  Data Type Conversion1 : DataTypeConversion  OutDataTypeStr=single
  Delay2 : Delay  DelayLength=sens_delay
      settings: AttributesFormatString=|
      | IC: %<InitialCondition>
      | Delay: %<DelayLength>
  Discrete-Time Integrator1 : DiscreteIntegrator  InitialCondition=single(0)  InitialConditionSetting=State (most efficient)  SampleTime=-1  ICPrevOutput=DiscIntNeverNeededParam  ICPrevScaledInput=DiscIntNeverNeededParam
      settings: AttributesFormatString=IC:%<InitialCondition>
  Gain1 : Gain  Gain=1/sqrt(sim_step_size)
  Gain3 : Gain  Gain=sens_sf
  Gain4 : Gain  Gain=1/sqrt(sim_step_size)
  Quantizer : Quantizer  QuantizationInterval=sens_resolution
  Saturation : Saturate  UpperLimit=sens_max  LowerLimit=sens_min
  Sum1 : Sum  Inputs=+++
  random_noise : RandomNumber  Variance=sens_sigma_u.^2  Seed=sens_rand_seed  SampleTime=sim_step_size
      settings: AttributesFormatString=|
      | Variance:%<Variance>
      | Mean:%<Mean>
      | Seed:%<Seed>
      | Sample Time:%<SampleTime>
  random_noise1 : RandomNumber  Variance=sens_sigma_v.^2  Seed=sens_rand_seed+1  SampleTime=sim_step_size
      settings: AttributesFormatString=|
      | Variance:%<Variance>
      | Mean:%<Mean>
      | Seed:%<Seed>
      | Sample Time:%<SampleTime>
  meas_speed : Outport
  wires:
  Data Type Conversion/1 -> Discrete-Time Integrator1/1
  Gain3/1 -> Sum1/1
  Data Type Conversion1/1 -> Sum1/2
  Discrete-Time Integrator1/1 -> Sum1/3
  Sum1/1 -> Quantizer/1
  Gain4/1 -> Data Type Conversion1/1
  Gain1/1 -> Data Type Conversion/1
  random_noise1/1 -> Gain1/1
  random_noise/1 -> Gain4/1
  truth_speed/1 -> Gain3/1
  Saturation/1 -> Delay2/1
  Delay2/1 -> meas_speed/1
  Quantizer/1 -> Saturation/1

== system util_generic_model_lib/dc_motor_model/dc_motor_model ==
  note: T_m = [(V- \omega*K_s)/R-i_o]*K_t - T_f
  note: Using negligible inductance formula from 'Comparison of Fixed and Variable Pitch Actuators for Agile Quadrotors'
  note: todo:
      | aero loading and dynamics
      | Stick-tion friction
  ctl_voltage : Inport
  curr_rotor_speed : Inport  Port=2
  Add : Sum  Inputs=+-
  Add1 : Sum  Inputs=+-
  Gain1 : Gain  Gain=motor_friction_coeff
  Gain4 : Gain  Gain=1/motor_kn
  Gain5 : Gain  Gain=1/motor_r
  Gain6 : Gain  Gain=motor_kt
  motor_torque : Outport
  motor_current : Outport  Port=2
  wires:
  Gain1/1 -> Add1/2  "viscous_friction"
  Add1/1 -> motor_torque/1  "output_torque"
  Gain6/1 -> Add1/1  "torque"
  Add/1 -> Gain5/1
  curr_rotor_speed/1 -> Gain4/1, Gain1/1
  Gain4/1 -> Add/2
  ctl_voltage/1 -> Add/1
  Gain5/1 -> motor_current/1, Gain6/1  "current"

== system util_generic_model_lib/dc_motor_model/speed_controller ==
  battery_voltage : Inport
  speed_cmd : Inport  Port=2
  speed_curr : Inport  Port=3
  Constant : Constant  Value=ctl_pwm2speed
  Discrete Transfer Fcn : DiscreteTransferFcn  Numerator=ctl_cmd_filt_num  Denominator=ctl_cmd_filt_den  SampleTime=controller_sample_time
      settings: AttributesFormatString=|
      | Num: %<Numerator>
      | Den: %<Denominator>
      | TS: %<SampleTime>
  Discrete Transfer Fcn1 : DiscreteTransferFcn  Numerator=ctl_speed_filt_num  Denominator=ctl_speed_cilt_den  SampleTime=controller_sample_time
      settings: AttributesFormatString=|
      | Num: %<Numerator>
      | Den: %<Denominator>
      | TS: %<SampleTime>
  Discrete PID Controller : simulink/Continuous/PID Controller  Controller=PID  TimeDomain=Discrete-time  SampleTime=controller_sample_time  IntegratorMethod=Forward Euler  FilterMethod=Forward Euler  Form=Parallel  UseFilter=on  ControllerParametersSource=internal  P=ctl_kp  I=ctl_ki  D=ctl_kd  N=ctl_filt_n  InitialConditionSource=internal  InitialConditionForIntegrator=0  InitialConditionForFilter=0  ExternalReset=none  LimitOutput=on  UpperSaturationLimit=ctl_max_voltage  LowerSaturationLimit=-ctl_max_voltage  LinearizeAsGain=off  AntiWindupMode=clamping  Kb=1  TrackingMode=off  Kt=1  PParamMin=[]  PParamMax=[]  IParamMin=[]  IParamMax=[]  DParamMin=[]  DParamMax=[]  NParamMin=[]  NParamMax=[]  KbParamMin=[]  KbParamMax=[]  KtParamMin=[]  KtParamMax=[]  POutMin=[]  POutMax=[]  IOutMin=[]  IOutMax=[]  DOutMin=[]  DOutMax=[]  NOutMin=[]  NOutMax=[]  KbOutMin=[]  KbOutMax=[]  KtOutMin=[]  KtOutMax=[]  IntegratorOutMin=[]  IntegratorOutMax=[]  FilterOutMin=[]  FilterOutMax=[]  SumOutMin=[]  SumOutMax=[]  SumI1OutMin=[]  SumI1OutMax=[]  SumI2OutMin=[]  SumI2OutMax=[]  SumI3OutMin=[]  SumI3OutMax=[]  SumDOutMin=[]  SumDOutMax=[]  SaturationOutMin=[]  SaturationOutMax=[]  IntegratorContinuousStateAttributes=''  IntegratorStateMustResolveToSignalObject=off  IntegratorRTWStateStorageClass=Auto  FilterContinuousStateAttributes=''  FilterStateMustResolveToSignalObject=off  FilterRTWStateStorageClass=Auto  DifferentiatorICPrevScaledInput=0  DifferentiatorOutMin=[]  DifferentiatorOutMax=[]
      settings: AttributesFormatString=|
      | Kp: %<P>
      | Ki: %<I>
      | Kd: %<D>
      | NFilt: %<N>
      | Ts: %<SampleTime>
      | 
      | min: %<LowerSaturationLimit>
      | max: %<UpperSaturationLimit>
  Divide : Product  Inputs=**
  Gain : Gain  Gain=-1
  Saturation Dynamic : simulink/Discontinuities/Saturation Dynamic  OutMin=[]  OutMax=[]  OutDataTypeStr=Inherit: Same as second input  OutDataType=fixdt(1, 16)  OutScaling=2^-10  DoSatur=off
  Sum : Sum  Inputs=+-
  motor_ctl_voltage : Outport
  wires:
  speed_cmd/1 -> Divide/1
  Constant/1 -> Divide/2
  Divide/1 -> Discrete Transfer Fcn/1
  Discrete Transfer Fcn/1 -> Sum/1
  Discrete Transfer Fcn1/1 -> Sum/2
  Saturation Dynamic/1 -> motor_ctl_voltage/1
  Sum/1 -> Discrete PID Controller/1
  speed_curr/1 -> Discrete Transfer Fcn1/1
  battery_voltage/1 -> Saturation Dynamic/1, [volt]
  Discrete PID Controller/1 -> Saturation Dynamic/2
  [volt] -> Gain/1
  Gain/1 -> Saturation Dynamic/3

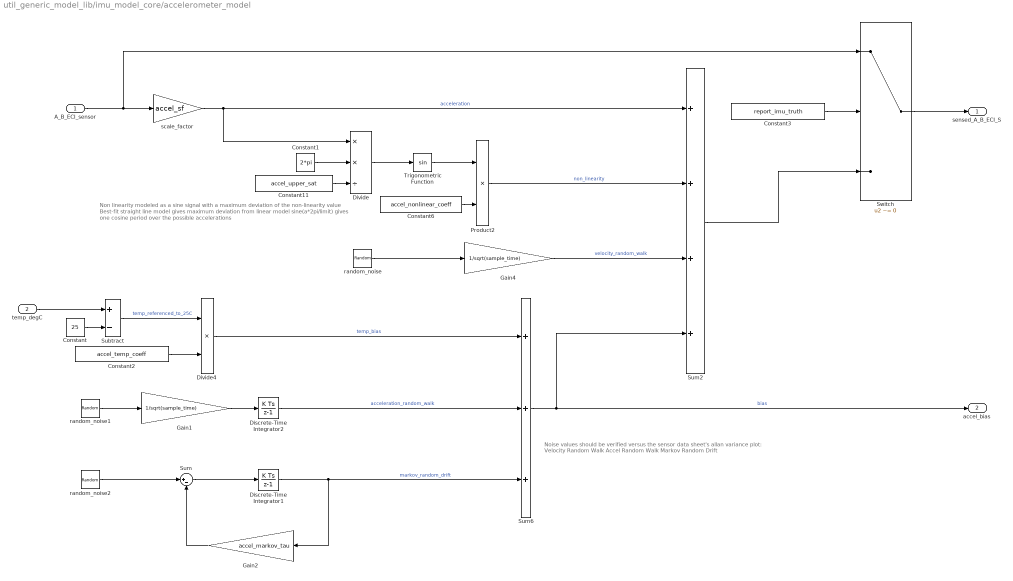
== system util_generic_model_lib/imu_model_core/accelerometer_model ==
  note: Non linearity modeled as a sine signal with a maximum deviation of the non-linearity value
      | Best-fit straight line model gives maximum deviation from linear model
      | sine(a*2pi/limit) gives one cosine period over the possible accelerations
  note: Noise values should be verified versus the sensor data sheet's allan variance plot:
      | Velocity Random Walk
      | Accel Random Walk
      | Markov Random Drift
  A_B_ECI_sensor : Inport
  temp_degC : Inport  Port=2
  Constant : Constant  Value=25
  Constant1 : Constant  Value=2*pi
  Constant11 : Constant  Value=accel_upper_sat
  Constant2 : Constant  Value=accel_temp_coeff
  Constant3 : Constant  Value=report_imu_truth
  Constant6 : Constant  Value=accel_nonlinear_coeff
  Discrete-Time Integrator1 : DiscreteIntegrator  InitialConditionSetting=State (most efficient)  SampleTime=-1  ICPrevOutput=DiscIntNeverNeededParam  ICPrevScaledInput=DiscIntNeverNeededParam
      settings: AttributesFormatString=IC:%<InitialCondition>
  Discrete-Time Integrator2 : DiscreteIntegrator  InitialCondition=accel_bias_ic  InitialConditionSetting=State (most efficient)  SampleTime=-1  ICPrevOutput=DiscIntNeverNeededParam  ICPrevScaledInput=DiscIntNeverNeededParam
      settings: AttributesFormatString=IC:%<InitialCondition>
  Divide : Product  Inputs=**/
  Divide4 : Product  Inputs=**
  Gain1 : Gain  Gain=1/sqrt(sample_time)
  Gain2 : Gain  Gain=accel_markov_tau
  Gain4 : Gain  Gain=1/sqrt(sample_time)
  Product2 : Product
  Subtract : Sum  Inputs=+-
  Sum : Sum  Inputs=|+-
  Sum2 : Sum  Inputs=++++
  Sum6 : Sum  Inputs=+++
  Switch : Switch  Criteria=u2 ~= 0
  Trigonometric Function : Trigonometry
  random_noise : RandomNumber  Variance=accel_sigma_vrw.^2  Seed=accel_noise_seed  SampleTime=sample_time
      settings: AttributesFormatString=|
      | Variance:%<Variance>
      | Mean:%<Mean>
      | Seed:%<Seed>
      | Sample Time:%<SampleTime>
  random_noise1 : RandomNumber  Variance=accel_sigma_arw.^2  Seed=accel_noise_seed+1  SampleTime=sample_time
      settings: AttributesFormatString=|
      | Variance:%<Variance>
      | Mean:%<Mean>
      | Seed:%<Seed>
      | Sample Time:%<SampleTime>
  random_noise2 : RandomNumber  Variance=accel_sigma_markov.^2  Seed=accel_noise_seed+2  SampleTime=sample_time
      settings: AttributesFormatString=|
      | Variance:%<Variance>
      | Mean:%<Mean>
      | Seed:%<Seed>
      | Sample Time:%<SampleTime>
  scale_factor : Gain  Gain=accel_sf
  sensed_A_B_ECI_S : Outport
  accel_bias : Outport  Port=2
  wires:
  A_B_ECI_sensor/1 -> scale_factor/1, Switch/1
  Sum2/1 -> Switch/3
  Constant3/1 -> Switch/2
  Gain2/1 -> Sum/2
  random_noise2/1 -> Sum/1
  Sum/1 -> Discrete-Time Integrator1/1
  Discrete-Time Integrator1/1 -> Gain2/1, Sum6/3  "markov_random_drift"
  temp_degC/1 -> Subtract/1
  Constant/1 -> Subtract/2
  Discrete-Time Integrator2/1 -> Sum6/2  "acceleration_random_walk"
  Gain4/1 -> Sum2/3  "velocity_random_walk"
  random_noise/1 -> Gain4/1
  random_noise1/1 -> Gain1/1
  Gain1/1 -> Discrete-Time Integrator2/1
  scale_factor/1 -> Sum2/1, Divide/1  "acceleration"
  Constant1/1 -> Divide/2
  Subtract/1 -> Divide4/1  "temp_referenced_to_25C"
  Constant2/1 -> Divide4/2
  Divide4/1 -> Sum6/1  "temp_bias"
  Constant6/1 -> Product2/2
  Constant11/1 -> Divide/3
  Trigonometric Function/1 -> Product2/1
  Divide/1 -> Trigonometric Function/1
  Product2/1 -> Sum2/2  "non_linearity"
  Sum6/1 -> accel_bias/1, Sum2/4  "bias"
  Switch/1 -> sensed_A_B_ECI_S/1

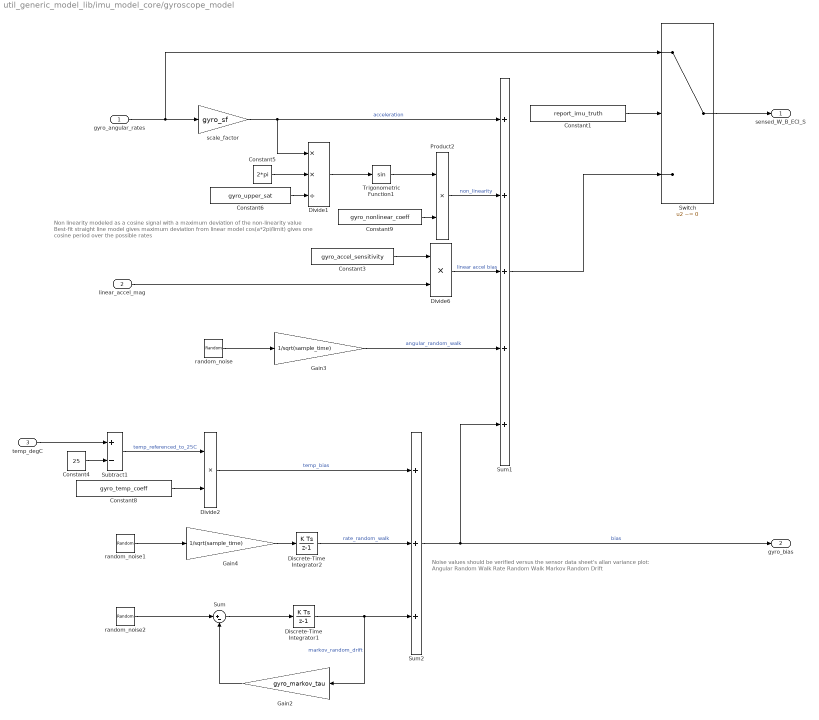
== system util_generic_model_lib/imu_model_core/gyroscope_model ==
  note: Non linearity modeled as a cosine signal with a maximum deviation of the non-linearity value
      | Best-fit straight line model gives maximum deviation from linear model
      | cos(a*2pi/limit) gives one cosine period over the possible rates
  note: Noise values should be verified versus the sensor data sheet's allan variance plot:
      | Angular Random Walk
      | Rate Random Walk
      | Markov Random Drift
  gyro_angular_rates : Inport
  linear_accel_mag : Inport  Port=2
  temp_degC : Inport  Port=3
  Constant1 : Constant  Value=report_imu_truth
  Constant3 : Constant  Value=gyro_accel_sensitivity
  Constant4 : Constant  Value=25
  Constant5 : Constant  Value=2*pi
  Constant6 : Constant  Value=gyro_upper_sat
  Constant8 : Constant  Value=gyro_temp_coeff
  Constant9 : Constant  Value=gyro_nonlinear_coeff
  Discrete-Time Integrator1 : DiscreteIntegrator  InitialConditionSetting=State (most efficient)  SampleTime=-1  ICPrevOutput=DiscIntNeverNeededParam  ICPrevScaledInput=DiscIntNeverNeededParam
      settings: AttributesFormatString=IC:%<InitialCondition>
  Discrete-Time Integrator2 : DiscreteIntegrator  InitialCondition=gyro_bias_ic  InitialConditionSetting=State (most efficient)  SampleTime=-1  ICPrevOutput=DiscIntNeverNeededParam  ICPrevScaledInput=DiscIntNeverNeededParam
      settings: AttributesFormatString=IC:%<InitialCondition>
  Divide1 : Product  Inputs=**/
  Divide2 : Product  Inputs=**
  Divide6 : Product  Inputs=**
  Gain2 : Gain  Gain=gyro_markov_tau
  Gain3 : Gain  Gain=1/sqrt(sample_time)
  Gain4 : Gain  Gain=1/sqrt(sample_time)
  Product2 : Product
  Subtract1 : Sum  Inputs=+-
  Sum : Sum  Inputs=|+-
  Sum1 : Sum  Inputs=+++++
  Sum2 : Sum  Inputs=+++
  Switch : Switch  Criteria=u2 ~= 0
  Trigonometric Function1 : Trigonometry
  random_noise : RandomNumber  Variance=gyro_sigma_arw.^2  Seed=gyro_noise_seed  SampleTime=sample_time
      settings: AttributesFormatString=|
      | Variance:%<Variance>
      | Mean:%<Mean>
      | Seed:%<Seed>
      | Sample Time:%<SampleTime>
  random_noise1 : RandomNumber  Variance=gyro_sigma_rrw.^2  Seed=gyro_noise_seed+1  SampleTime=sample_time
      settings: AttributesFormatString=|
      | Variance:%<Variance>
      | Mean:%<Mean>
      | Seed:%<Seed>
      | Sample Time:%<SampleTime>
  random_noise2 : RandomNumber  Variance=gyro_sigma_markov.^2  Seed=gyro_noise_seed+2  SampleTime=sample_time
      settings: AttributesFormatString=|
      | Variance:%<Variance>
      | Mean:%<Mean>
      | Seed:%<Seed>
      | Sample Time:%<SampleTime>
  scale_factor : Gain  Gain=gyro_sf
  sensed_W_B_ECI_S : Outport
  gyro_bias : Outport  Port=2
  wires:
  Sum1/1 -> Switch/3
  Constant1/1 -> Switch/2
  Switch/1 -> sensed_W_B_ECI_S/1
  Gain2/1 -> Sum/2
  random_noise2/1 -> Sum/1
  Sum/1 -> Discrete-Time Integrator1/1
  Discrete-Time Integrator1/1 -> Sum2/3, Gain2/1  "markov_random_drift"
  temp_degC/1 -> Subtract1/1
  Constant4/1 -> Subtract1/2
  Discrete-Time Integrator2/1 -> Sum2/2  "rate_random_walk"
  Gain3/1 -> Sum1/4  "angular_random_walk"
  random_noise/1 -> Gain3/1
  random_noise1/1 -> Gain4/1
  Gain4/1 -> Discrete-Time Integrator2/1
  scale_factor/1 -> Sum1/1, Divide1/1  "acceleration"
  gyro_angular_rates/1 -> scale_factor/1, Switch/1
  Constant5/1 -> Divide1/2
  Subtract1/1 -> Divide2/1  "temp_referenced_to_25C"
  Constant8/1 -> Divide2/2
  Divide2/1 -> Sum2/1  "temp_bias"
  Constant9/1 -> Product2/2
  Constant6/1 -> Divide1/3
  Trigonometric Function1/1 -> Product2/1
  Divide1/1 -> Trigonometric Function1/1
  Product2/1 -> Sum1/2  "non_linearity"
  Divide6/1 -> Sum1/3  "linear accel bias"
  linear_accel_mag/1 -> Divide6/2
  Constant3/1 -> Divide6/1
  Sum2/1 -> gyro_bias/1, Sum1/5  "bias"

== system util_generic_model_lib/imu_model_core/imu_hardware ==
  sensable_accel : Inport
  sensable_rate : Inport  Port=2
  Delay1 : Delay  DelayLength=imu_output_delay
      settings: AttributesFormatString=|
      | IC: %<InitialCondition>
      | Delay: %<DelayLength>
  Delay2 : Delay  DelayLength=imu_output_delay
      settings: AttributesFormatString=|
      | IC: %<InitialCondition>
      | Delay: %<DelayLength>
  Discrete Transfer Fcn : DiscreteTransferFcn  Numerator=gyro_filter_num  Denominator=gyro_filter_den
      settings: AttributesFormatString=|
      | Num: %<Numerator>
      | Den: %<Denominator>
  Discrete Transfer Fcn1 : DiscreteTransferFcn  Numerator=accel_filter_num  Denominator=accel_filter_den
      settings: AttributesFormatString=|
      | Num: %<Numerator>
      | Den: %<Denominator>
  Quantizer : Quantizer  QuantizationInterval=accel_resolution
  Quantizer1 : Quantizer  QuantizationInterval=gyro_resolution
  Saturation : Saturate  UpperLimit=accel_upper_sat  LowerLimit=accel_lower_sat
  Saturation1 : Saturate  UpperLimit=gyro_upper_sat  LowerLimit=gyro_lower_sat
  accel_output : Outport
  rate_output : Outport  Port=2
  wires:
  Discrete Transfer Fcn/1 -> Quantizer1/1
  Discrete Transfer Fcn1/1 -> Quantizer/1
  Delay2/1 -> accel_output/1
  Saturation1/1 -> Delay1/1
  Delay1/1 -> rate_output/1
  Saturation/1 -> Delay2/1
  sensable_accel/1 -> Discrete Transfer Fcn1/1
  sensable_rate/1 -> Discrete Transfer Fcn/1
  Quantizer/1 -> Saturation/1
  Quantizer1/1 -> Saturation1/1

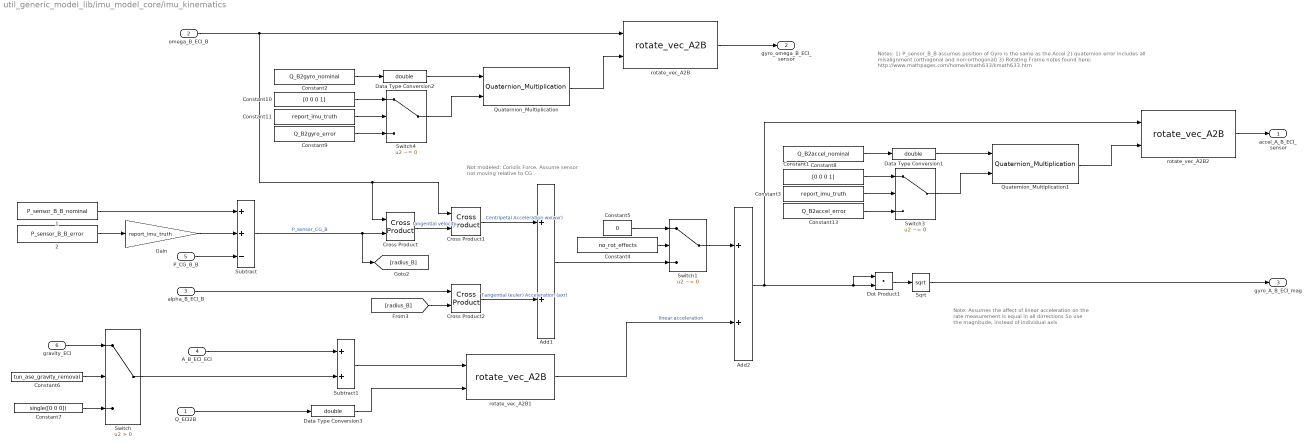
== system util_generic_model_lib/imu_model_core/imu_kinematics ==
  note: Note: Assumes the affect of linear acceleration
      | on the rate measurement is equal in all dirrections
      | So use the magnitude, instead of individual axis
  note: Not modeled: Coriolis Force.
      | Assume sensor not moving relative to CG
  note: Notes:
      | 	1) P_sensor_B_B assumes position of Gyro is the same as the Accel
      | 	2) quaternion error includes all misalignment (orthogonal and non-orthogonal)
      | 	3) Rotating Frame notes found here: http://www.mathpages.com/home/kmath633/kmath633.htm
  Q_ECI2B : Inport
  omega_B_ECI_B : Inport  Port=2
  alpha_B_ECI_B : Inport  Port=3
  A_B_ECI_ECI : Inport  Port=4
  P_CG_B_B : Inport  Port=5
  gravity_ECI : Inport  Port=6
  " 1" : Constant  Value=P_sensor_B_B_nominal
  " 2" : Constant  Value=P_sensor_B_B_error
  Add1 : Sum
  Add2 : Sum
  Constant1 : Constant  Value=[0 0 0 1]
  Constant10 : Constant  Value=[0 0 0 1]
  Constant11 : Constant  Value=report_imu_truth
  Constant13 : Constant  Value=Q_B2accel_error
  Constant2 : Constant  Value=Q_B2gyro_nominal
  Constant3 : Constant  Value=report_imu_truth
  Constant4 : Constant  Value=no_rot_effects
  Constant5 : Constant  Value=0
  Constant6 : Constant  Value=tun_ase_gravity_removal
  Constant7 : Constant  Value=single([0 0 0])
  Constant8 : Constant  Value=Q_B2accel_nominal
  Constant9 : Constant  Value=Q_B2gyro_error
  Cross Product : vrlib/Utilities/Cross Product
  Cross Product1 : vrlib/Utilities/Cross Product
  Cross Product2 : vrlib/Utilities/Cross Product
  Data Type Conversion1 : DataTypeConversion  OutDataTypeStr=double
  Data Type Conversion2 : DataTypeConversion  OutDataTypeStr=double
  Data Type Conversion3 : DataTypeConversion  OutDataTypeStr=double
  Dot Product1 : DotProduct  InputSameDT=on  OutDataTypeStr=Inherit: Inherit via internal rule
  Gain : Gain  Gain=report_imu_truth
  Quaternion_Multiplication : math_utils/Quaternion_Multiplication  SystemSampleTime=-1
  Quaternion_Multiplication1 : math_utils/Quaternion_Multiplication  SystemSampleTime=-1
  Sqrt : Sqrt  SaturateOnIntegerOverflow=on
  Subtract : Sum  Inputs=++-
  Subtract1 : Sum
  Switch : Switch  Criteria=u2 > Threshold
  Switch1 : Switch  Criteria=u2 ~= 0
  Switch3 : Switch  Criteria=u2 ~= 0
  Switch4 : Switch  Criteria=u2 ~= 0
  rotate_vec_A2B : math_utils/rotate_vec_A2B  SystemSampleTime=-1
  rotate_vec_A2B1 : math_utils/rotate_vec_A2B  SystemSampleTime=-1
  rotate_vec_A2B2 : math_utils/rotate_vec_A2B  SystemSampleTime=-1
  accel_A_B_ECI_sensor : Outport
  gyro_omega_B_ECI_sensor : Outport  Port=2
  gyro_A_B_ECI_mag : Outport  Port=3
  wires:
  rotate_vec_A2B2/1 -> accel_A_B_ECI_sensor/1
  Add2/1 -> rotate_vec_A2B2/1, Dot Product1/2, Dot Product1/1
  Constant5/1 -> Switch1/1
  Add1/1 -> Switch1/3
  Switch1/1 -> Add2/1
  Constant4/1 -> Switch1/2
  rotate_vec_A2B/1 -> gyro_omega_B_ECI_sensor/1
  Constant2/1 -> Data Type Conversion2/1
  omega_B_ECI_B/1 -> rotate_vec_A2B/1, Cross Product1/1, Cross Product/1
  " 1"/1 -> Subtract/1
  P_CG_B_B/1 -> Subtract/3
  rotate_vec_A2B1/1 -> Add2/2  "linear acceleration"
  Subtract1/1 -> rotate_vec_A2B1/1
  A_B_ECI_ECI/1 -> Subtract1/1
  Q_ECI2B/1 -> Data Type Conversion3/1
  Sqrt/1 -> gyro_A_B_ECI_mag/1
  Dot Product1/1 -> Sqrt/1
  [radius_B] -> Cross Product2/2
  alpha_B_ECI_B/1 -> Cross Product2/1
  Subtract/1 -> Cross Product/2, [radius_B]  "P_sensor_CG_B"
  Cross Product2/1 -> Add1/2  "Tangential (euler) Acceleration (axr)"
  Cross Product1/1 -> Add1/1  "Centripetal Acceleration wx(wxr)"
  Cross Product/1 -> Cross Product1/2  "tangential velocity"
  Data Type Conversion2/1 -> Quaternion_Multiplication/1
  Data Type Conversion3/1 -> rotate_vec_A2B1/2
  Constant10/1 -> Switch4/1
  Constant9/1 -> Switch4/3
  Constant11/1 -> Switch4/2
  Switch4/1 -> Quaternion_Multiplication/2
  Quaternion_Multiplication/1 -> rotate_vec_A2B/2
  Constant8/1 -> Data Type Conversion1/1
  Data Type Conversion1/1 -> Quaternion_Multiplication1/1
  Constant1/1 -> Switch3/1
  Constant13/1 -> Switch3/3
  Constant3/1 -> Switch3/2
  Switch3/1 -> Quaternion_Multiplication1/2
  Quaternion_Multiplication1/1 -> rotate_vec_A2B2/2
  " 2"/1 -> Gain/1
  Gain/1 -> Subtract/2
  Constant7/1 -> Switch/3
  Constant6/1 -> Switch/2
  gravity_ECI/1 -> Switch/1
  Switch/1 -> Subtract1/2
